simulink model "gm_InterlockDeadtime3L"  (R2025b)
settings: Solver=FixedStepDiscrete  StartTime=0.0  StopTime=0.0000004  RelTol=1e-3
undefined symbols (not defined in the file or in its folder): T_FPGA_clk
libraries: simulink x4, hdlsllib x4
settings Model: PacingRate=0.010000  Creator=info  LastModifiedBy=info
settings OptimizationCC: BlockReduction=off  ConditionallyExecuteInputs=off  DefaultParameterBehavior=Inlined
settings DebuggingCC: AlgebraicLoopMsg=error  InheritedTsInSrcMsg=none
settings HardwareCC: ProdBitPerPointer=32.0  ProdBitPerSizeT=32.0  ProdBitPerPtrDiffT=32.0  ProdLargestAtomicFloat=None  ProdIntDivRoundTo=Undefined  ProdEndianess=Unspecified  ProdWordSize=32.0  ProdHWDeviceType=ASIC/FPGA->ASIC/FPGA  TargetBitPerPointer=64.0  TargetBitPerSizeT=64.0  TargetBitPerPtrDiffT=64.0  TargetLongLongMode=on  TargetIntDivRoundTo=Zero  TargetEndianess=LittleEndian  TargetWordSize=64.0  TargetHWDeviceType=Custom Processor->MATLAB Host Computer  ProdEqTarget=off

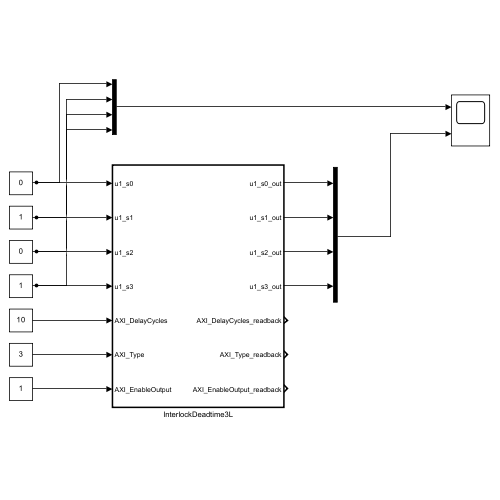
[thumbnail: Simulink's stored preview of the top-level diagram]
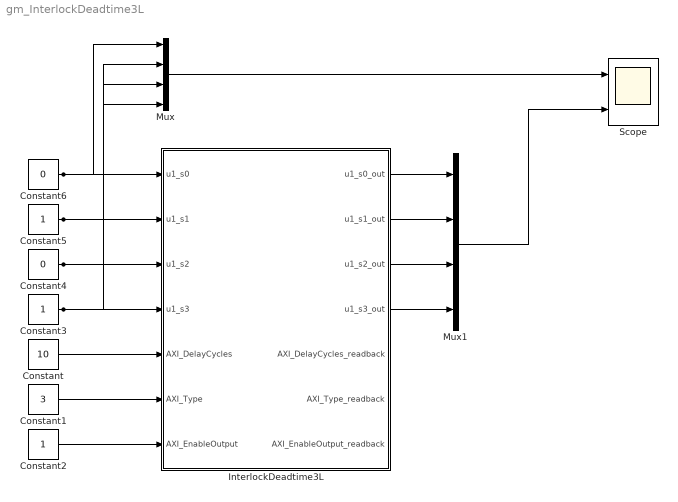
== system gm_InterlockDeadtime3L ==
  Constant : Constant  Value=10  OutDataTypeStr=uint32  SampleTime=T_FPGA_clk
  Constant1 : Constant  Value=3  OutDataTypeStr=uint8  SampleTime=T_FPGA_clk
  Constant2 : Constant  OutDataTypeStr=boolean  SampleTime=T_FPGA_clk
  Constant3 : Constant  OutDataTypeStr=boolean  SampleTime=T_FPGA_clk
  Constant4 : Constant  Value=0  OutDataTypeStr=boolean  SampleTime=T_FPGA_clk
  Constant5 : Constant  OutDataTypeStr=boolean  SampleTime=T_FPGA_clk
  Constant6 : Constant  Value=0  OutDataTypeStr=boolean  SampleTime=T_FPGA_clk
  InterlockDeadtime3L : Subsystem  TreatAsAtomicUnit=on
  Mux : Mux
  Mux1 : Mux
  Scope : Scope  NumInputPorts=2
      settings: ActiveDisplayYMinimum=-0.12499999999999997  ActiveDisplayYMaximum=1.125  DataLoggingVariableName=ScopeData2  DataLoggingSaveFormat=Array
  wires:
  Mux1/1 -> Scope/2
  InterlockDeadtime3L/4(u1_s3_out) -> Mux1/4
  InterlockDeadtime3L/3(u1_s2_out) -> Mux1/3
  InterlockDeadtime3L/2(u1_s1_out) -> Mux1/2
  InterlockDeadtime3L/1(u1_s0_out) -> Mux1/1
  Mux/1 -> Scope/1
  Constant4/1 -> InterlockDeadtime3L/3(u1_s2), Mux/3
  Constant5/1 -> InterlockDeadtime3L/2(u1_s1), Mux/2
  Constant6/1 -> Mux/1, InterlockDeadtime3L/1(u1_s0)
  Constant3/1 -> InterlockDeadtime3L/4(u1_s3), Mux/4
  Constant2/1 -> InterlockDeadtime3L/7(AXI_EnableOutput)
  Constant1/1 -> InterlockDeadtime3L/6(AXI_Type)
  Constant/1 -> InterlockDeadtime3L/5(AXI_DelayCycles)

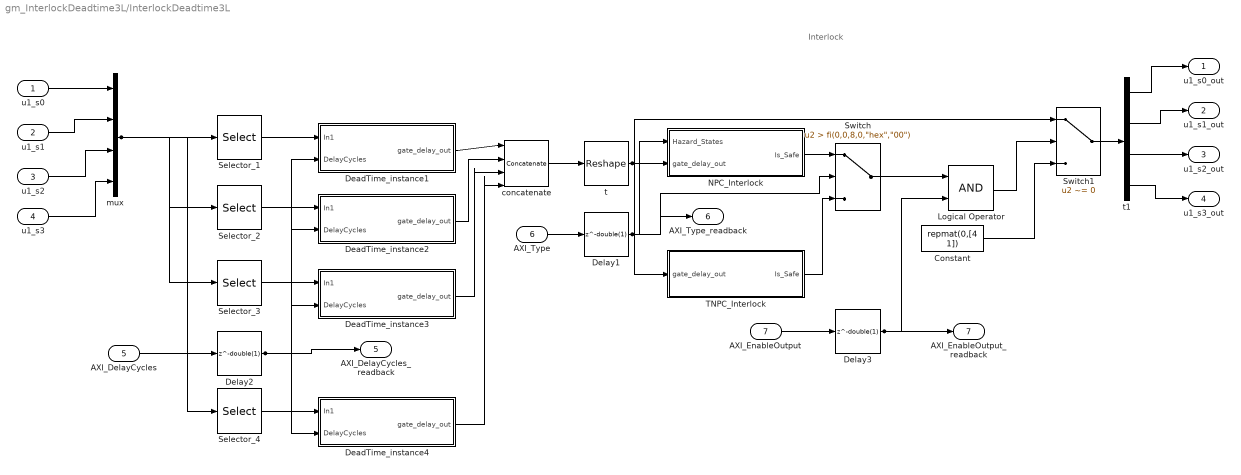
== system gm_InterlockDeadtime3L/InterlockDeadtime3L ==
  note: Interlock
  u1_s0 : Inport  OutDataTypeStr=boolean  PortDimensions=1  SampleTime=1e-08
  u1_s1 : Inport  Port=2  OutDataTypeStr=boolean  PortDimensions=1  SampleTime=1e-08
  u1_s2 : Inport  Port=3  OutDataTypeStr=boolean  PortDimensions=1  SampleTime=1e-08
  u1_s3 : Inport  Port=4  OutDataTypeStr=boolean  PortDimensions=1  SampleTime=1e-08
  AXI_DelayCycles : Inport  Port=5  OutDataTypeStr=uint32  PortDimensions=1  SampleTime=1e-08
  AXI_Type : Inport  Port=6  OutDataTypeStr=uint8  PortDimensions=1  SampleTime=1e-08
  AXI_EnableOutput : Inport  Port=7  OutDataTypeStr=boolean  PortDimensions=1  SampleTime=1e-08
  Constant : Constant  Value="repmat(0,[4  1])"  OutDataTypeStr=boolean  SampleTime=1e-08
  DeadTime_instance1 : Subsystem
  DeadTime_instance2 : Subsystem
  DeadTime_instance3 : Subsystem
  DeadTime_instance4 : Subsystem
  Delay1 : Delay  DelayLength=double(1)  InitialCondition=0  SampleTime=1e-08
  Delay2 : Delay  DelayLength=double(1)  InitialCondition=0  SampleTime=1e-08
  Delay3 : Delay  DelayLength=double(1)  InitialCondition=0  SampleTime=1e-08
  Logical Operator : Logic  AllPortsSameDT=off  OutDataTypeStr=boolean  SampleTime=1e-08
  NPC_Interlock : Subsystem
  Selector_1 : Selector  InputPortWidth=4  IndexOptions=Index vector (dialog)  Indices=double(1)  OutputSizes=1
  Selector_2 : Selector  InputPortWidth=4  IndexOptions=Index vector (dialog)  Indices=double(2)  OutputSizes=1
  Selector_3 : Selector  InputPortWidth=4  IndexOptions=Index vector (dialog)  Indices=double(3)  OutputSizes=1
  Selector_4 : Selector  InputPortWidth=4  IndexOptions=Index vector (dialog)  Indices=double(4)  OutputSizes=1
  Switch : Switch  Criteria=u2 > Threshold  Threshold="fi(0,0,8,0,\"hex\",\"00\")"  OutDataTypeStr=boolean  SampleTime=1e-08  SaturateOnIntegerOverflow=off  InputSameDT=off
  Switch1 : Switch  Criteria=u2 ~= 0  Threshold="fi(0,0,1,0,\"hex\",\"0\")"  OutDataTypeStr=boolean  SampleTime=1e-08  SaturateOnIntegerOverflow=off  InputSameDT=off
  TNPC_Interlock : Subsystem
  concatenate : Concatenate  NumInputs=4
  mux : Mux
  t : Reshape
  t1 : Demux
  u1_s0_out : Outport  OutDataTypeStr=boolean  SampleTime=1e-08  VectorParamsAs1DForOutWhenUnconnected=off
  u1_s1_out : Outport  Port=2  OutDataTypeStr=boolean  SampleTime=1e-08  VectorParamsAs1DForOutWhenUnconnected=off
  u1_s2_out : Outport  Port=3  OutDataTypeStr=boolean  SampleTime=1e-08  VectorParamsAs1DForOutWhenUnconnected=off
  u1_s3_out : Outport  Port=4  OutDataTypeStr=boolean  SampleTime=1e-08  VectorParamsAs1DForOutWhenUnconnected=off
  AXI_DelayCycles_readback : Outport  Port=5  SampleTime=1e-08
  AXI_Type_readback : Outport  Port=6  SampleTime=1e-08
  AXI_EnableOutput_readback : Outport  Port=7  SampleTime=1e-08
  wires:
  u1_s0/1 -> mux/1
  u1_s1/1 -> mux/2
  t1/1 -> u1_s0_out/1
  u1_s2/1 -> mux/3
  u1_s3/1 -> mux/4
  mux/1 -> Selector_4/1, Selector_2/1, Selector_1/1, Selector_3/1
  AXI_DelayCycles/1 -> Delay2/1
  Selector_2/1 -> DeadTime_instance2/1(In1)
  Selector_1/1 -> DeadTime_instance1/1(In1)
  Selector_3/1 -> DeadTime_instance3/1(In1)
  Delay3/1 -> Logical Operator/2, AXI_EnableOutput_readback/1
  Delay2/1 -> DeadTime_instance4/2(DelayCycles), DeadTime_instance2/2(DelayCycles), DeadTime_instance1/2(DelayCycles), DeadTime_instance3/2(DelayCycles), AXI_DelayCycles_readback/1
  Selector_4/1 -> DeadTime_instance4/1(In1)
  DeadTime_instance1/1(gate_delay_out) -> concatenate/1
  AXI_EnableOutput/1 -> Delay3/1
  DeadTime_instance2/1(gate_delay_out) -> concatenate/2
  DeadTime_instance3/1(gate_delay_out) -> concatenate/3
  DeadTime_instance4/1(gate_delay_out) -> concatenate/4
  concatenate/1 -> t/1
  AXI_Type/1 -> Delay1/1
  t/1 -> Switch1/1, NPC_Interlock/2(gate_delay_out), TNPC_Interlock/1(gate_delay_out)
  Delay1/1 -> Switch/2, NPC_Interlock/1(Hazard_States), AXI_Type_readback/1
  NPC_Interlock/1(Is_Safe) -> Switch/1
  TNPC_Interlock/1(Is_Safe) -> Switch/3
  Switch/1 -> Logical Operator/1
  Logical Operator/1 -> Switch1/2
  Constant/1 -> Switch1/3
  Switch1/1 -> t1/1
  t1/4 -> u1_s3_out/1
  t1/3 -> u1_s2_out/1
  t1/2 -> u1_s1_out/1

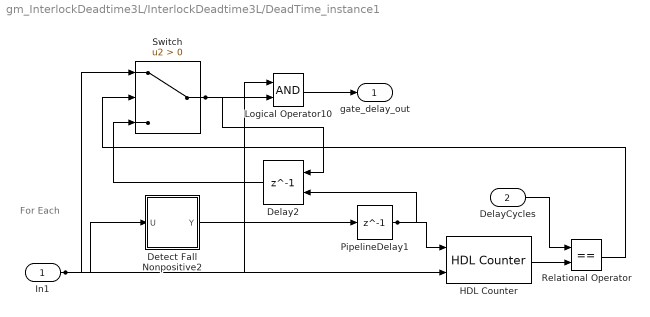
== system gm_InterlockDeadtime3L/InterlockDeadtime3L/DeadTime_instance1 ==
  note: For Each
  In1 : Inport  OutDataTypeStr=boolean  PortDimensions=1  SampleTime=1e-08
  DelayCycles : Inport  Port=2  OutDataTypeStr=uint32  PortDimensions=1  SampleTime=1e-08
  Delay2 : Delay  DelayLength=1  ExternalReset=Level  UseCircularBuffer=on
      settings: InputPortMap=u0,r5
  Detect Fall Nonpositive2 : Subsystem  mask(Detect Fall Nonpositive){vinit=double(0), InputProcessing=Elements as channels (sample based), OutDataTypeStr=boolean}
      mask prompts: vinit "Simulink:masks:InitialCondition_MP"; InputProcessing "Simulink:masks:InputProcessing_MP"; OutDataTypeStr "Simulink:masks:OutputDataType_MP"
      mask help: Simulink:masks:DetectFallNonpositive_MD
      mask init:
      | InputProcessing = 'Elements as channels (sample based)';
      | OutDataTypeStr = 'boolean';
      | vinit = double(0);
      mask TypeOptions InputProcessing: Simulink:masks:ColumnsAsChannelsFrameBased | Simulink:masks:ElementsAsChannelsSampleBased
      mask TypeOptions OutDataTypeStr: Simulink:masks:uint8 | Simulink:masks:boolean
      mask Display: fprintf('U <= 0\n&  NOT\nU/z <= 0')
  HDL Counter : hdlsllib/Sources/HDL Counter  CountType=Free running  CountInit=0  CountStep=1  CountMax=25  CountFromType=Initial value  CountFrom=0  CountResetPort=on  CountLoadPort=off  CountEnbPort=on  CountDirPort=off  CountHitOutputPort=off  CountDataType=Unsigned  CountWordLen=10  CountFracLen=0  CountSampTime=-1
  Logical Operator10 : Logic  AllPortsSameDT=off  OutDataTypeStr=boolean
  PipelineDelay1 : Delay  DelayLength=1
  Relational Operator : RelationalOperator  Operator===  OutDataTypeStr=boolean  RndMeth=Simplest  InputSameDT=off
  Switch : Switch  Criteria=u2 > Threshold  OutDataTypeStr=boolean  SaturateOnIntegerOverflow=off  InputSameDT=off
  gate_delay_out : Outport  SampleTime=1e-08
  wires:
  In1/1 -> Logical Operator10/1, HDL Counter/2, Switch/1, Detect Fall Nonpositive2/1(U)
  Delay2/1 -> Switch/3
  Switch/1 -> Delay2/1, Logical Operator10/2
  Logical Operator10/1 -> gate_delay_out/1
  Detect Fall Nonpositive2/1(Y) -> PipelineDelay1/1
  DelayCycles/1 -> Relational Operator/1
  PipelineDelay1/1 -> Delay2/2, HDL Counter/1
  HDL Counter/1 -> Relational Operator/2
  Relational Operator/1 -> Switch/2

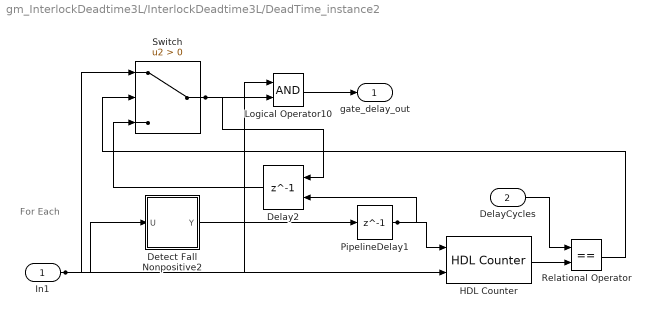
== system gm_InterlockDeadtime3L/InterlockDeadtime3L/DeadTime_instance2 ==
  note: For Each
  In1 : Inport  OutDataTypeStr=boolean  PortDimensions=1  SampleTime=1e-08
  DelayCycles : Inport  Port=2  OutDataTypeStr=uint32  PortDimensions=1  SampleTime=1e-08
  Delay2 : Delay  DelayLength=1  ExternalReset=Level  UseCircularBuffer=on
      settings: InputPortMap=u0,r5
  Detect Fall Nonpositive2 : Subsystem  mask(Detect Fall Nonpositive){vinit=double(0), InputProcessing=Elements as channels (sample based), OutDataTypeStr=boolean}
      mask prompts: vinit "Simulink:masks:InitialCondition_MP"; InputProcessing "Simulink:masks:InputProcessing_MP"; OutDataTypeStr "Simulink:masks:OutputDataType_MP"
      mask help: Simulink:masks:DetectFallNonpositive_MD
      mask init:
      | InputProcessing = 'Elements as channels (sample based)';
      | OutDataTypeStr = 'boolean';
      | vinit = double(0);
      mask TypeOptions InputProcessing: Simulink:masks:ColumnsAsChannelsFrameBased | Simulink:masks:ElementsAsChannelsSampleBased
      mask TypeOptions OutDataTypeStr: Simulink:masks:uint8 | Simulink:masks:boolean
      mask Display: fprintf('U <= 0\n&  NOT\nU/z <= 0')
  HDL Counter : hdlsllib/Sources/HDL Counter  CountType=Free running  CountInit=0  CountStep=1  CountMax=25  CountFromType=Initial value  CountFrom=0  CountResetPort=on  CountLoadPort=off  CountEnbPort=on  CountDirPort=off  CountHitOutputPort=off  CountDataType=Unsigned  CountWordLen=10  CountFracLen=0  CountSampTime=-1
  Logical Operator10 : Logic  AllPortsSameDT=off  OutDataTypeStr=boolean
  PipelineDelay1 : Delay  DelayLength=1
  Relational Operator : RelationalOperator  Operator===  OutDataTypeStr=boolean  RndMeth=Simplest  InputSameDT=off
  Switch : Switch  Criteria=u2 > Threshold  OutDataTypeStr=boolean  SaturateOnIntegerOverflow=off  InputSameDT=off
  gate_delay_out : Outport  SampleTime=1e-08
  wires:
  In1/1 -> HDL Counter/2, Switch/1, Detect Fall Nonpositive2/1(U), Logical Operator10/1
  HDL Counter/1 -> Relational Operator/2
  DelayCycles/1 -> Relational Operator/1
  Switch/1 -> Delay2/1, Logical Operator10/2
  Delay2/1 -> Switch/3
  Detect Fall Nonpositive2/1(Y) -> PipelineDelay1/1
  Logical Operator10/1 -> gate_delay_out/1
  PipelineDelay1/1 -> Delay2/2, HDL Counter/1
  Relational Operator/1 -> Switch/2

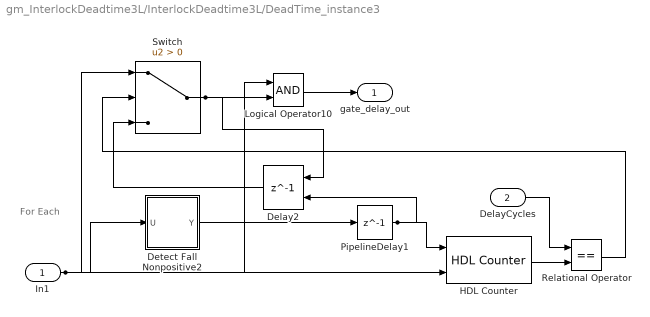
== system gm_InterlockDeadtime3L/InterlockDeadtime3L/DeadTime_instance3 ==
  note: For Each
  In1 : Inport  OutDataTypeStr=boolean  PortDimensions=1  SampleTime=1e-08
  DelayCycles : Inport  Port=2  OutDataTypeStr=uint32  PortDimensions=1  SampleTime=1e-08
  Delay2 : Delay  DelayLength=1  ExternalReset=Level  UseCircularBuffer=on
      settings: InputPortMap=u0,r5
  Detect Fall Nonpositive2 : Subsystem  mask(Detect Fall Nonpositive){vinit=double(0), InputProcessing=Elements as channels (sample based), OutDataTypeStr=boolean}
      mask prompts: vinit "Simulink:masks:InitialCondition_MP"; InputProcessing "Simulink:masks:InputProcessing_MP"; OutDataTypeStr "Simulink:masks:OutputDataType_MP"
      mask help: Simulink:masks:DetectFallNonpositive_MD
      mask init:
      | InputProcessing = 'Elements as channels (sample based)';
      | OutDataTypeStr = 'boolean';
      | vinit = double(0);
      mask TypeOptions InputProcessing: Simulink:masks:ColumnsAsChannelsFrameBased | Simulink:masks:ElementsAsChannelsSampleBased
      mask TypeOptions OutDataTypeStr: Simulink:masks:uint8 | Simulink:masks:boolean
      mask Display: fprintf('U <= 0\n&  NOT\nU/z <= 0')
  HDL Counter : hdlsllib/Sources/HDL Counter  CountType=Free running  CountInit=0  CountStep=1  CountMax=25  CountFromType=Initial value  CountFrom=0  CountResetPort=on  CountLoadPort=off  CountEnbPort=on  CountDirPort=off  CountHitOutputPort=off  CountDataType=Unsigned  CountWordLen=10  CountFracLen=0  CountSampTime=-1
  Logical Operator10 : Logic  AllPortsSameDT=off  OutDataTypeStr=boolean
  PipelineDelay1 : Delay  DelayLength=1
  Relational Operator : RelationalOperator  Operator===  OutDataTypeStr=boolean  RndMeth=Simplest  InputSameDT=off
  Switch : Switch  Criteria=u2 > Threshold  OutDataTypeStr=boolean  SaturateOnIntegerOverflow=off  InputSameDT=off
  gate_delay_out : Outport  SampleTime=1e-08
  wires:
  Switch/1 -> Delay2/1, Logical Operator10/2
  In1/1 -> Logical Operator10/1, HDL Counter/2, Switch/1, Detect Fall Nonpositive2/1(U)
  Detect Fall Nonpositive2/1(Y) -> PipelineDelay1/1
  DelayCycles/1 -> Relational Operator/1
  Delay2/1 -> Switch/3
  HDL Counter/1 -> Relational Operator/2
  Logical Operator10/1 -> gate_delay_out/1
  PipelineDelay1/1 -> Delay2/2, HDL Counter/1
  Relational Operator/1 -> Switch/2

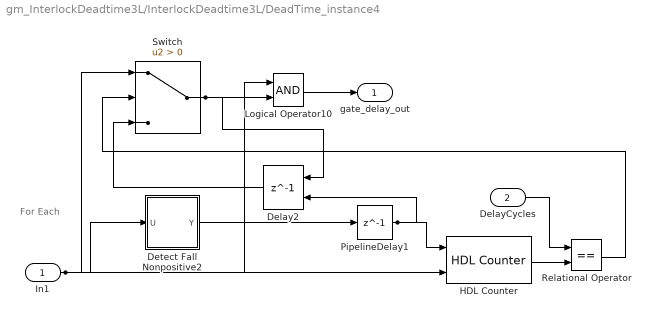
== system gm_InterlockDeadtime3L/InterlockDeadtime3L/DeadTime_instance4 ==
  note: For Each
  In1 : Inport  OutDataTypeStr=boolean  PortDimensions=1  SampleTime=1e-08
  DelayCycles : Inport  Port=2  OutDataTypeStr=uint32  PortDimensions=1  SampleTime=1e-08
  Delay2 : Delay  DelayLength=1  ExternalReset=Level  UseCircularBuffer=on
      settings: InputPortMap=u0,r5
  Detect Fall Nonpositive2 : Subsystem  mask(Detect Fall Nonpositive){vinit=double(0), InputProcessing=Elements as channels (sample based), OutDataTypeStr=boolean}
      mask prompts: vinit "Simulink:masks:InitialCondition_MP"; InputProcessing "Simulink:masks:InputProcessing_MP"; OutDataTypeStr "Simulink:masks:OutputDataType_MP"
      mask help: Simulink:masks:DetectFallNonpositive_MD
      mask init:
      | InputProcessing = 'Elements as channels (sample based)';
      | OutDataTypeStr = 'boolean';
      | vinit = double(0);
      mask TypeOptions InputProcessing: Simulink:masks:ColumnsAsChannelsFrameBased | Simulink:masks:ElementsAsChannelsSampleBased
      mask TypeOptions OutDataTypeStr: Simulink:masks:uint8 | Simulink:masks:boolean
      mask Display: fprintf('U <= 0\n&  NOT\nU/z <= 0')
  HDL Counter : hdlsllib/Sources/HDL Counter  CountType=Free running  CountInit=0  CountStep=1  CountMax=25  CountFromType=Initial value  CountFrom=0  CountResetPort=on  CountLoadPort=off  CountEnbPort=on  CountDirPort=off  CountHitOutputPort=off  CountDataType=Unsigned  CountWordLen=10  CountFracLen=0  CountSampTime=-1
  Logical Operator10 : Logic  AllPortsSameDT=off  OutDataTypeStr=boolean
  PipelineDelay1 : Delay  DelayLength=1
  Relational Operator : RelationalOperator  Operator===  OutDataTypeStr=boolean  RndMeth=Simplest  InputSameDT=off
  Switch : Switch  Criteria=u2 > Threshold  OutDataTypeStr=boolean  SaturateOnIntegerOverflow=off  InputSameDT=off
  gate_delay_out : Outport  SampleTime=1e-08
  wires:
  In1/1 -> HDL Counter/2, Switch/1, Logical Operator10/1, Detect Fall Nonpositive2/1(U)
  Logical Operator10/1 -> gate_delay_out/1
  Delay2/1 -> Switch/3
  Switch/1 -> Logical Operator10/2, Delay2/1
  Detect Fall Nonpositive2/1(Y) -> PipelineDelay1/1
  PipelineDelay1/1 -> HDL Counter/1, Delay2/2
  DelayCycles/1 -> Relational Operator/1
  HDL Counter/1 -> Relational Operator/2
  Relational Operator/1 -> Switch/2

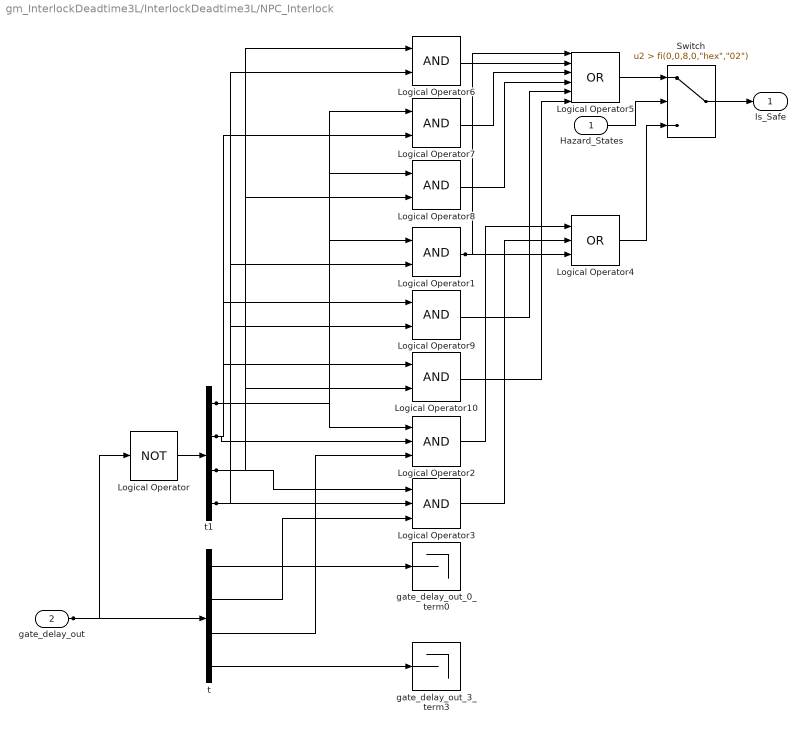
== system gm_InterlockDeadtime3L/InterlockDeadtime3L/NPC_Interlock ==
  Hazard_States : Inport  OutDataTypeStr=uint8  PortDimensions=1  SampleTime=1e-08
  gate_delay_out : Inport  Port=2  OutDataTypeStr=boolean  PortDimensions=[4]  SampleTime=1e-08
  Logical Operator : Logic  Operator=NOT  Inputs=1  AllPortsSameDT=off  OutDataTypeStr=boolean  SampleTime=1e-08
  Logical Operator{1,6..10} (6 alike) : Logic  AllPortsSameDT=off  OutDataTypeStr=boolean  SampleTime=1e-08
  Logical Operator2 : Logic  Inputs=3  AllPortsSameDT=off  OutDataTypeStr=boolean  SampleTime=1e-08
  Logical Operator3 : Logic  Inputs=3  AllPortsSameDT=off  OutDataTypeStr=boolean  SampleTime=1e-08
  Logical Operator4 : Logic  Operator=OR  Inputs=3  AllPortsSameDT=off  OutDataTypeStr=boolean  SampleTime=1e-08
  Logical Operator5 : Logic  Operator=OR  Inputs=6  AllPortsSameDT=off  OutDataTypeStr=boolean  SampleTime=1e-08
  Switch : Switch  Criteria=u2 > Threshold  Threshold="fi(0,0,8,0,\"hex\",\"02\")"  OutDataTypeStr=boolean  SampleTime=1e-08  SaturateOnIntegerOverflow=off  InputSameDT=off
  gate_delay_out_0_term0 : Terminator
  gate_delay_out_3_term3 : Terminator
  t : Demux
  t1 : Demux
  Is_Safe : Outport  SampleTime=1e-08
  wires:
  gate_delay_out/1 -> t/1, Logical Operator/1
  Logical Operator1/1 -> Logical Operator5/1, Logical Operator4/3
  Logical Operator/1 -> t1/1
  t1/1 -> Logical Operator8/1, Logical Operator2/1, Logical Operator1/1, Logical Operator7/1
  t1/2 -> Logical Operator9/1, Logical Operator7/2, Logical Operator2/2, Logical Operator10/1
  t1/3 -> Logical Operator6/1, Logical Operator3/1, Logical Operator10/2, Logical Operator8/2
  t1/4 -> Logical Operator9/2, Logical Operator3/2, Logical Operator6/2, Logical Operator1/2
  t/1 -> gate_delay_out_0_term0/1
  t/4 -> gate_delay_out_3_term3/1
  t/3 -> Logical Operator2/3
  t/2 -> Logical Operator3/3
  Logical Operator6/1 -> Logical Operator5/2
  Logical Operator7/1 -> Logical Operator5/3
  Logical Operator8/1 -> Logical Operator5/4
  Logical Operator9/1 -> Logical Operator5/5
  Logical Operator10/1 -> Logical Operator5/6
  Logical Operator2/1 -> Logical Operator4/1
  Logical Operator3/1 -> Logical Operator4/2
  Logical Operator5/1 -> Switch/1
  Hazard_States/1 -> Switch/2
  Logical Operator4/1 -> Switch/3
  Switch/1 -> Is_Safe/1

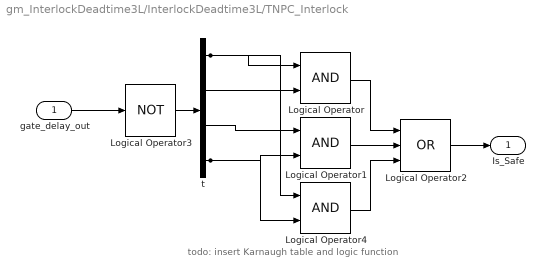
== system gm_InterlockDeadtime3L/InterlockDeadtime3L/TNPC_Interlock ==
  note: todo: insert Karnaugh table and logic function
  gate_delay_out : Inport  OutDataTypeStr=boolean  PortDimensions=[4]  SampleTime=1e-08
  Logical Operator : Logic  AllPortsSameDT=off  OutDataTypeStr=boolean  SampleTime=1e-08
  Logical Operator1 : Logic  AllPortsSameDT=off  OutDataTypeStr=boolean  SampleTime=1e-08
  Logical Operator2 : Logic  Operator=OR  Inputs=3  AllPortsSameDT=off  OutDataTypeStr=boolean  SampleTime=1e-08
  Logical Operator3 : Logic  Operator=NOT  Inputs=1  AllPortsSameDT=off  OutDataTypeStr=boolean  SampleTime=1e-08
  Logical Operator4 : Logic  AllPortsSameDT=off  OutDataTypeStr=boolean  SampleTime=1e-08
  t : Demux
  Is_Safe : Outport  SampleTime=1e-08
  wires:
  gate_delay_out/1 -> Logical Operator3/1
  Logical Operator3/1 -> t/1
  Logical Operator/1 -> Logical Operator2/1
  t/1 -> Logical Operator4/1, Logical Operator/1
  t/2 -> Logical Operator/2
  Logical Operator1/1 -> Logical Operator2/2
  t/3 -> Logical Operator1/1
  t/4 -> Logical Operator4/2, Logical Operator1/2
  Logical Operator4/1 -> Logical Operator2/3
  Logical Operator2/1 -> Is_Safe/1

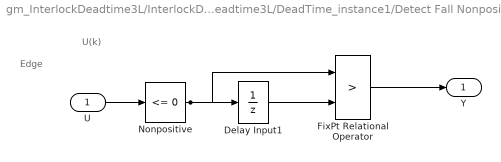
== system gm_InterlockDeadtime3L/InterlockDeadtime3L/DeadTime_instance1/Detect Fall Nonpositive2 ==
  note: U(k)
  note: Edge
  U : Inport  OutDataTypeStr=boolean  SampleTime=1e-08
  Delay Input1 : UnitDelay  Description=Store in Global RAM  DisableCoverage=on  InitialCondition=vinit  SampleTime=-1  HasFrameUpgradeWarning=on
  FixPt Relational Operator : RelationalOperator  Operator=>  OutDataTypeStr=boolean  ZeroCross=off  InputSameDT=off
  Nonpositive : simulink/Logic and Bit Operations/Compare To Zero  relop=<=  OutDataTypeStr=boolean  ZeroCross=off
  Y : Outport  SampleTime=1e-08  InitialOutput=0
  wires:
  U/1 -> Nonpositive/1
  Nonpositive/1 -> FixPt Relational Operator/1, Delay Input1/1
  Delay Input1/1 -> FixPt Relational Operator/2
  FixPt Relational Operator/1 -> Y/1

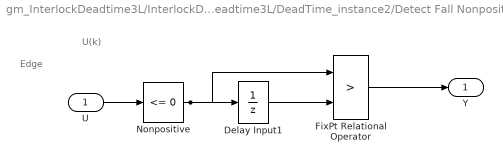
== system gm_InterlockDeadtime3L/InterlockDeadtime3L/DeadTime_instance2/Detect Fall Nonpositive2 ==
  note: Edge
  note: U(k)
  U : Inport  OutDataTypeStr=boolean  SampleTime=1e-08
  Delay Input1 : UnitDelay  Description=Store in Global RAM  DisableCoverage=on  InitialCondition=vinit  SampleTime=-1  HasFrameUpgradeWarning=on
  FixPt Relational Operator : RelationalOperator  Operator=>  OutDataTypeStr=boolean  ZeroCross=off  InputSameDT=off
  Nonpositive : simulink/Logic and Bit Operations/Compare To Zero  relop=<=  OutDataTypeStr=boolean  ZeroCross=off
  Y : Outport  SampleTime=1e-08  InitialOutput=0
  wires:
  FixPt Relational Operator/1 -> Y/1
  Delay Input1/1 -> FixPt Relational Operator/2
  Nonpositive/1 -> Delay Input1/1, FixPt Relational Operator/1
  U/1 -> Nonpositive/1

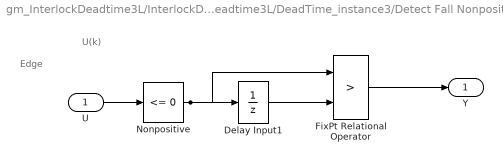
== system gm_InterlockDeadtime3L/InterlockDeadtime3L/DeadTime_instance3/Detect Fall Nonpositive2 ==
  note: Edge
  note: U(k)
  U : Inport  OutDataTypeStr=boolean  SampleTime=1e-08
  Delay Input1 : UnitDelay  Description=Store in Global RAM  DisableCoverage=on  InitialCondition=vinit  SampleTime=-1  HasFrameUpgradeWarning=on
  FixPt Relational Operator : RelationalOperator  Operator=>  OutDataTypeStr=boolean  ZeroCross=off  InputSameDT=off
  Nonpositive : simulink/Logic and Bit Operations/Compare To Zero  relop=<=  OutDataTypeStr=boolean  ZeroCross=off
  Y : Outport  SampleTime=1e-08  InitialOutput=0
  wires:
  FixPt Relational Operator/1 -> Y/1
  Delay Input1/1 -> FixPt Relational Operator/2
  Nonpositive/1 -> Delay Input1/1, FixPt Relational Operator/1
  U/1 -> Nonpositive/1

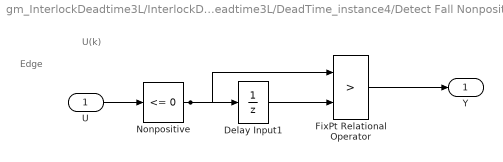
== system gm_InterlockDeadtime3L/InterlockDeadtime3L/DeadTime_instance4/Detect Fall Nonpositive2 ==
  note: Edge
  note: U(k)
  U : Inport  OutDataTypeStr=boolean  SampleTime=1e-08
  Delay Input1 : UnitDelay  Description=Store in Global RAM  DisableCoverage=on  InitialCondition=vinit  SampleTime=-1  HasFrameUpgradeWarning=on
  FixPt Relational Operator : RelationalOperator  Operator=>  OutDataTypeStr=boolean  ZeroCross=off  InputSameDT=off
  Nonpositive : simulink/Logic and Bit Operations/Compare To Zero  relop=<=  OutDataTypeStr=boolean  ZeroCross=off
  Y : Outport  SampleTime=1e-08  InitialOutput=0
  wires:
  FixPt Relational Operator/1 -> Y/1
  Delay Input1/1 -> FixPt Relational Operator/2
  Nonpositive/1 -> Delay Input1/1, FixPt Relational Operator/1
  U/1 -> Nonpositive/1
